simulink library "CryoDetLibCMB"  (R2016b)
settings: Solver=VariableStepAuto  StartTime=0.0  StopTime=10.0  RelTol=1e-3
undefined symbols (not defined in the file): Fclk, xlipgetpartsetting
libraries: xbsIndex_r4 x329, CryoDetLibCMB x20, CryoDetLib x2, simulink x1
(part 3 of 3)

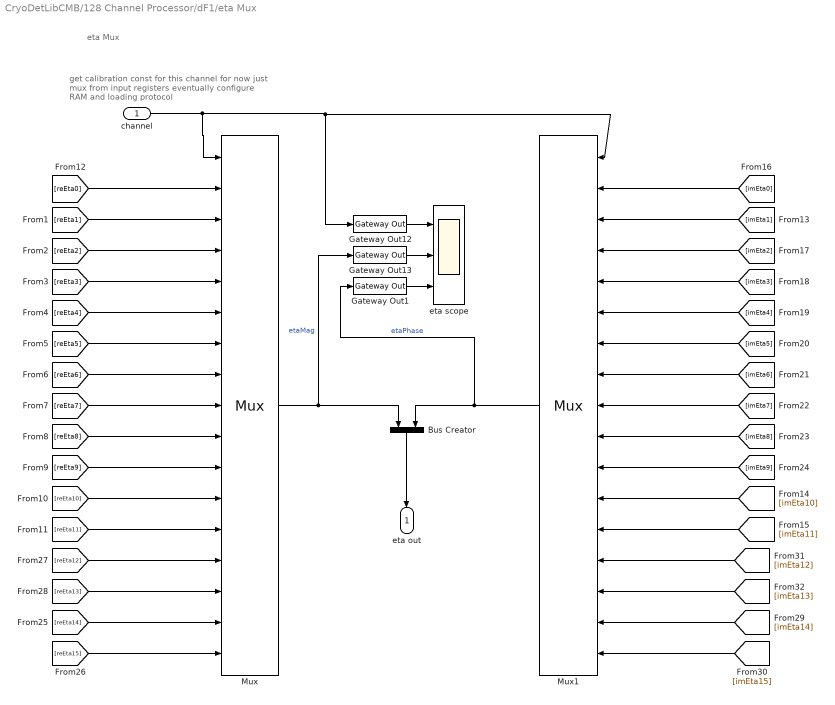
== system CryoDetLibCMB/128 Channel Processor/dF1/eta Mux ==
  note: eta Mux
  note: get calibration const for this channel
      | for now just mux from input registers
      | eventually configure RAM and loading protocol
  channel : Inport
  Bus Creator : BusCreator  Inputs=2
  Gateway Out1 : xbsIndex_r4/Gateway Out  inherit_from_input=off  hdl_port=off  rows=1  columns=1  UseAsDAC=off  DACChannel='1'  interface=None  automatic_assignment=on  address_offset=hex2dec('00')  intf_name=''  intf_description=''  timing_constraint=None  locs_specified=off  LOCs={}  io_standard={}  block_type=gatewayout
  Gateway Out12 : xbsIndex_r4/Gateway Out  inherit_from_input=off  hdl_port=off  rows=1  columns=1  UseAsDAC=off  DACChannel='1'  interface=None  automatic_assignment=on  address_offset=hex2dec('00')  intf_name=''  intf_description=''  timing_constraint=None  locs_specified=off  LOCs={}  io_standard={}  block_type=gatewayout
  Gateway Out13 : xbsIndex_r4/Gateway Out  inherit_from_input=off  hdl_port=off  rows=1  columns=1  UseAsDAC=off  DACChannel='1'  interface=None  automatic_assignment=on  address_offset=hex2dec('00')  intf_name=''  intf_description=''  timing_constraint=None  locs_specified=off  LOCs={}  io_standard={}  block_type=gatewayout
  Mux : xbsIndex_r4/Mux  inputs=16  en=off  latency=1  precision=Full  arith_type=Unsigned  n_bits=24  bin_pt=24  quantization=Truncate  overflow=Wrap  dbl_ovrd=off  block_type=mux
  Mux1 : xbsIndex_r4/Mux  inputs=16  en=off  latency=1  precision=Full  arith_type=Unsigned  n_bits=24  bin_pt=24  quantization=Truncate  overflow=Wrap  dbl_ovrd=off  block_type=mux
  eta scope : Scope  NumInputPorts=3
  eta out : Outport
  wires:
  channel/1 -> Mux/1, Gateway Out12/1, Mux1/1
  [reEta0] -> Mux/2
  [reEta1] -> Mux/3
  [reEta2] -> Mux/4
  [reEta3] -> Mux/5
  [reEta4] -> Mux/6
  [reEta5] -> Mux/7
  [reEta6] -> Mux/8
  [reEta7] -> Mux/9
  [reEta8] -> Mux/10
  [reEta9] -> Mux/11
  [reEta10] -> Mux/12
  [reEta11] -> Mux/13
  Mux/1 -> Bus Creator/1, Gateway Out13/1  "etaMag"
  Gateway Out13/1 -> eta scope/2
  Gateway Out12/1 -> eta scope/1
  [imEta0] -> Mux1/2
  [imEta1] -> Mux1/3
  [imEta2] -> Mux1/4
  [imEta3] -> Mux1/5
  [imEta4] -> Mux1/6
  [imEta5] -> Mux1/7
  [imEta6] -> Mux1/8
  [imEta7] -> Mux1/9
  [imEta8] -> Mux1/10
  [imEta9] -> Mux1/11
  [imEta10] -> Mux1/12
  [imEta11] -> Mux1/13
  Mux1/1 -> Bus Creator/2, Gateway Out1/1  "etaPhase"
  Gateway Out1/1 -> eta scope/3
  Bus Creator/1 -> eta out/1
  [reEta15] -> Mux/17
  [reEta14] -> Mux/16
  [reEta13] -> Mux/15
  [reEta12] -> Mux/14
  [imEta12] -> Mux1/14
  [imEta13] -> Mux1/15
  [imEta14] -> Mux1/16
  [imEta15] -> Mux1/17

== system CryoDetLibCMB/128 Channel Processor/dF1/ref phase RAM ==
  ref Phase : Inport
  read channel : Inport  Port=2
  Bus Creator1 : BusCreator  Inputs=2
  Bus Selector5 : BusSelector  OutputSignals=channel,refPhase
  Delay1 : xbsIndex_r4/Delay  rst=off  infoeditControl=Selection of Reset will increase slice count due to use of real FFs and instead of SRLs  en=off  latency=1  reg_retiming=off  dbl_ovrd=off  block_type=delay
  Dual Port RAM : xbsIndex_r4/Dual Port RAM  depth=16  initVector=0  distributed_mem=Distributed memory  init_a=0  init_b=0  rst_a=off  rst_b=off  en_a=off  en_b=off  latency=1  write_mode_A=Read Before Write  write_mode_B=Read After Write  optimize=Area  dbl_ovrd=off  block_type=dpram
  Terminator : Terminator
  write : xbsIndex_r4/Constant  const=1.0  gui_display_data_type=Boolean  arith_type=Boolean  n_bits=16  bin_pt=14  preci_type=Single  exp_width=8  frac_width=24  explicit_period=off  period=1  equ=P=C  opselect=C  inp2=PCIN>>17  opr=+  inp1=P  carry=CIN  dbl_ovrd=off  block_type=constant
  ref phase : Outport
  wires:
  write/1 -> Dual Port RAM/3
  Delay1/1 -> Bus Creator1/1  "chan"
  Dual Port RAM/2 -> Bus Creator1/2  "ref phase"
  Bus Creator1/1 -> ref phase/1
  read channel/1 -> Dual Port RAM/4, Delay1/1
  Dual Port RAM/1 -> Terminator/1
  ref Phase/1 -> Bus Selector5/1
  Bus Selector5/1 -> Dual Port RAM/1  "<channel>"
  Bus Selector5/2 -> Dual Port RAM/2  "<refPhase>"

== system CryoDetLibCMB/128 Channel Processor/dF1/ref phase diff ==
  note: ref phase diff
      | calulates difference in phase between present phase of DDS generating tone for a resonator and its phase when the signal now being recieved was generated.
      | That is this pahse difference is the integral of the frequency history of the tone generaotr over the ADC/DAC/cable/cryo latency
  note: ref delay is ADC/DAC/cryo latency in units of Fclk/16
  ref phase : Inport
  AddSub : xbsIndex_r4/AddSub  mode=Subtraction  use_carryin=off  use_carryout=off  en=off  latency=1  precision=Full  arith_type=Unsigned  n_bits=16  bin_pt=14  quantization=Truncate  overflow=Wrap  use_behavioral_HDL=off  hw_selection=Fabric  pipelined=off  dbl_ovrd=off  block_type=addsub
  Addressable Shift Register : xbsIndex_r4/Addressable Shift Register  infer_latency=on  depth=2  initVector=[0]  en=off  use_behavioral_HDL=off  Optimization=Resource  dbl_ovrd=off  block_type=addrsr
      settings: infoedit="Delay of configurable length.  Any element in the delay line can be addressed and driven onto the output port.<br><br>Hardware notes: Generates fast, compact FIFO-style shift registers or delay lines using SRL16/SRL32 mode of the slice LUTs"
  Bus Creator2 : BusCreator  Inputs=2
  Bus Selector5 : BusSelector  OutputSignals=channel,DDS Ref
  Delay : xbsIndex_r4/Delay  rst=off  infoeditControl=Selection of Reset will increase slice count due to use of real FFs and instead of SRLs  en=off  latency=1  reg_retiming=off  dbl_ovrd=off  block_type=delay
  Delay2 : xbsIndex_r4/Delay  rst=off  infoeditControl=Selection of Reset will increase slice count due to use of real FFs and instead of SRLs  en=off  latency=1  reg_retiming=off  dbl_ovrd=off  block_type=delay
  Shift : xbsIndex_r4/Shift  shift_dir=Left  shift_bits=4  en=off  latency=0  precision=User Defined  arith_type=Unsigned  n_bits=8  bin_pt=0  quantization=Truncate  overflow=Wrap  dbl_ovrd=off  block_type=shift
  phase diff : Outport
  wires:
  ref phase/1 -> Bus Selector5/1
  [refDel] -> Shift/1
  Shift/1 -> Addressable Shift Register/2
  Addressable Shift Register/1 -> AddSub/2
  Bus Selector5/2 -> AddSub/1, Addressable Shift Register/1  "<DDS Ref>"
  Delay/1 -> Delay2/1
  Bus Selector5/1 -> Delay/1  "<channel>"
  Delay2/1 -> Bus Creator2/1  "channel"
  AddSub/1 -> Bus Creator2/2  "refPhase"
  Bus Creator2/1 -> phase diff/1

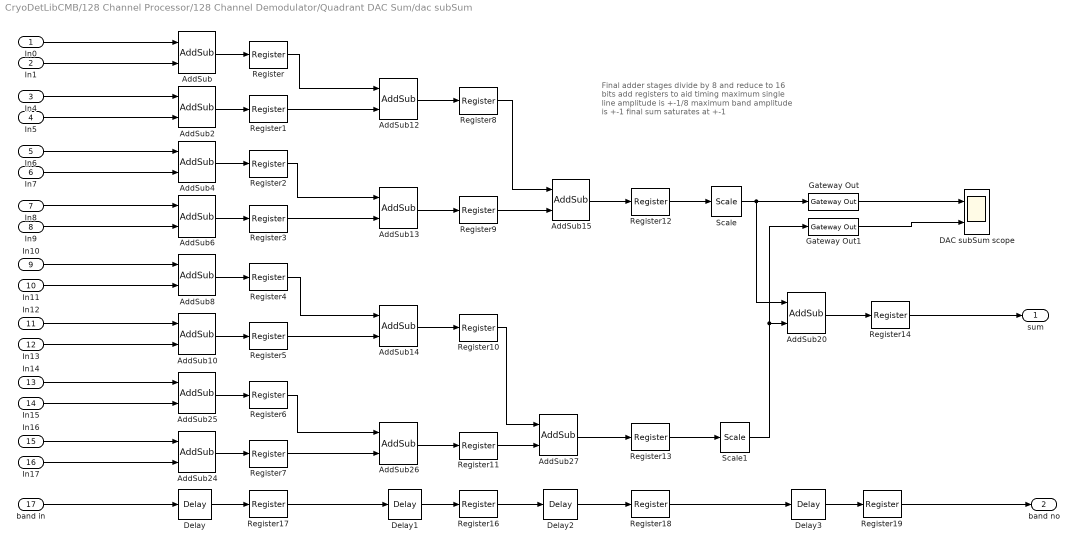
== system CryoDetLibCMB/128 Channel Processor/128 Channel Demodulator/Quadrant DAC Sum/dac subSum ==
  note: Final adder stages
      | divide by 8
      | and reduce to 16 bits
      | add registers to aid timing
      | maximum single line amplitude is +-1/8
      | maximum band amplitude is +-1
      | final sum saturates at +-1
  In0 : Inport
  In1 : Inport  Port=2
  In4 : Inport  Port=3
  In5 : Inport  Port=4
  In6 : Inport  Port=5
  In7 : Inport  Port=6
  In8 : Inport  Port=7
  In9 : Inport  Port=8
  In10 : Inport  Port=9
  In11 : Inport  Port=10
  In12 : Inport  Port=11
  In13 : Inport  Port=12
  In14 : Inport  Port=13
  In15 : Inport  Port=14
  In16 : Inport  Port=15
  In17 : Inport  Port=16
  band in : Inport  Port=17
  AddSub{,2,4,8,10,12..14,24..26} (11 alike) : xbsIndex_r4/AddSub  mode=Addition  use_carryin=off  use_carryout=off  en=off  latency=3  precision=User Defined  arith_type="Signed  (2's comp)"  n_bits=20  bin_pt=17  quantization=Truncate  overflow=Wrap  use_behavioral_HDL=off  hw_selection=Fabric  pipelined=off  dbl_ovrd=off  block_type=addsub
  AddSub15 : xbsIndex_r4/AddSub  mode=Addition  use_carryin=off  use_carryout=off  en=off  latency=3  precision=User Defined  arith_type="Signed  (2's comp)"  n_bits=21  bin_pt=17  quantization=Truncate  overflow=Wrap  use_behavioral_HDL=off  hw_selection=Fabric  pipelined=off  dbl_ovrd=off  block_type=addsub
  AddSub20 : xbsIndex_r4/AddSub  mode=Addition  use_carryin=off  use_carryout=off  en=off  latency=3  precision=User Defined  arith_type="Signed  (2's comp)"  n_bits=21  bin_pt=20  quantization=Truncate  overflow=Saturate  use_behavioral_HDL=off  hw_selection=Fabric  pipelined=off  dbl_ovrd=off  block_type=addsub
  AddSub27 : xbsIndex_r4/AddSub  mode=Addition  use_carryin=off  use_carryout=off  en=off  latency=3  precision=User Defined  arith_type="Signed  (2's comp)"  n_bits=21  bin_pt=17  quantization=Truncate  overflow=Wrap  use_behavioral_HDL=off  hw_selection=Fabric  pipelined=off  dbl_ovrd=off  block_type=addsub
  AddSub6 : xbsIndex_r4/AddSub  mode=Addition  use_carryin=off  use_carryout=off  en=off  latency=3  precision=User Defined  arith_type="Signed  (2's comp)"  n_bits=20  bin_pt=15  quantization=Truncate  overflow=Wrap  use_behavioral_HDL=off  hw_selection=Fabric  pipelined=off  dbl_ovrd=off  block_type=addsub
  DAC subSum scope : Scope  NumInputPorts=2
  Delay{,1..3} (4 alike) : xbsIndex_r4/Delay  rst=off  infoeditControl=Selection of Reset will increase slice count due to use of real FFs and instead of SRLs  en=off  latency=3  reg_retiming=on  dbl_ovrd=off  block_type=delay
  Gateway Out : xbsIndex_r4/Gateway Out  inherit_from_input=off  hdl_port=off  rows=1  columns=1  UseAsDAC=off  DACChannel='1'  interface=None  automatic_assignment=on  address_offset=hex2dec('00')  intf_name=''  intf_description=''  timing_constraint=None  locs_specified=off  LOCs={}  io_standard={}  block_type=gatewayout
  Gateway Out1 : xbsIndex_r4/Gateway Out  inherit_from_input=off  hdl_port=off  rows=1  columns=1  UseAsDAC=off  DACChannel='1'  interface=None  automatic_assignment=on  address_offset=hex2dec('00')  intf_name=''  intf_description=''  timing_constraint=None  locs_specified=off  LOCs={}  io_standard={}  block_type=gatewayout
  Register{,1..14,16..19} (19 alike) : xbsIndex_r4/Register  init=0  rst=off  en=off  dbl_ovrd=off  block_type=register
  Scale : xbsIndex_r4/Scale  scale_factor=-3  dbl_ovrd=off  block_type=scale
  Scale1 : xbsIndex_r4/Scale  scale_factor=-3  dbl_ovrd=off  block_type=scale
  sum : Outport
  band no : Outport  Port=2
  wires:
  Register14/1 -> sum/1
  Register13/1 -> Scale1/1
  Register12/1 -> Scale/1
  Register11/1 -> AddSub27/2
  Register10/1 -> AddSub27/1
  Register9/1 -> AddSub15/2
  Register8/1 -> AddSub15/1
  Register7/1 -> AddSub26/2
  Register6/1 -> AddSub26/1
  Register5/1 -> AddSub14/2
  Register4/1 -> AddSub14/1
  Register3/1 -> AddSub13/2
  Register2/1 -> AddSub13/1
  Register1/1 -> AddSub12/2
  Register/1 -> AddSub12/1
  Gateway Out/1 -> DAC subSum scope/1
  Gateway Out1/1 -> DAC subSum scope/2
  In9/1 -> AddSub6/2
  In1/1 -> AddSub/2
  In4/1 -> AddSub2/1
  In5/1 -> AddSub2/2
  In6/1 -> AddSub4/1
  In7/1 -> AddSub4/2
  In8/1 -> AddSub6/1
  In10/1 -> AddSub8/1
  In11/1 -> AddSub8/2
  In12/1 -> AddSub10/1
  In13/1 -> AddSub10/2
  In14/1 -> AddSub25/1
  In15/1 -> AddSub25/2
  In16/1 -> AddSub24/1
  In17/1 -> AddSub24/2
  AddSub26/1 -> Register11/1
  AddSub27/1 -> Register13/1
  AddSub14/1 -> Register10/1
  AddSub24/1 -> Register7/1
  AddSub25/1 -> Register6/1
  Scale1/1 -> AddSub20/2, Gateway Out1/1
  Scale/1 -> AddSub20/1, Gateway Out/1
  AddSub15/1 -> Register12/1
  AddSub13/1 -> Register9/1
  AddSub12/1 -> Register8/1
  AddSub10/1 -> Register5/1
  AddSub8/1 -> Register4/1
  AddSub6/1 -> Register3/1
  AddSub4/1 -> Register2/1
  AddSub2/1 -> Register1/1
  AddSub/1 -> Register/1
  AddSub20/1 -> Register14/1
  In0/1 -> AddSub/1
  Delay/1 -> Register17/1
  band in/1 -> Delay/1
  Register17/1 -> Delay1/1
  Delay1/1 -> Register16/1
  Register16/1 -> Delay2/1
  Delay2/1 -> Register18/1
  Register18/1 -> Delay3/1
  Delay3/1 -> Register19/1
  Register19/1 -> band no/1
